simulink model "W1P6"  (R2020b)
settings: Solver=VariableStepAuto  StartTime=0.0  StopTime=10.0  RelTol=1e-3
settings Model: Creator=Dell  LastModifiedBy=Dell

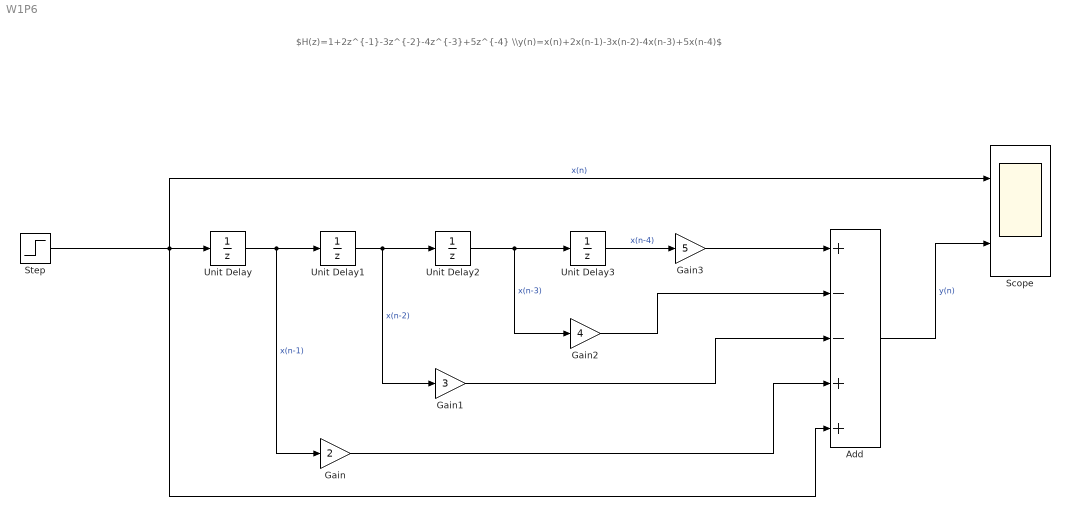
== system W1P6 ==
  note: $H(z)=1+2z^{-1}-3z^{-2}-4z^{-3}+5z^{-4} \\y(n)=x(n)+2x(n-1)-3x(n-2)-4x(n-3)+5x(n-4)$
  Add : Sum  Inputs=+--++
  Gain : Gain  Gain=2
  Gain1 : Gain  Gain=3
  Gain2 : Gain  Gain=4
  Gain3 : Gain  Gain=5
  Scope : Scope  NumInputPorts=2
  Step : Step  SampleTime=0
  Unit Delay{,1..3} (4 alike) : UnitDelay  InitialCondition=0.1  SampleTime=-1  HasFrameUpgradeWarning=on
  wires:
  Unit Delay/1 -> Gain/1, Unit Delay1/1  "x(n-1)"
  Unit Delay1/1 -> Gain1/1, Unit Delay2/1  "x(n-2)"
  Unit Delay2/1 -> Gain2/1, Unit Delay3/1  "x(n-3)"
  Unit Delay3/1 -> Gain3/1  "x(n-4)"
  Gain2/1 -> Add/2
  Gain3/1 -> Add/1
  Gain1/1 -> Add/3
  Gain/1 -> Add/4
  Step/1 -> Scope/1, Add/5, Unit Delay/1  "x(n)"
  Add/1 -> Scope/2  "y(n)"
